simulink model "stellaris_helloworld"  (R2013a)
settings: Solver=FixedStepDiscrete  SolverMode=SingleTasking  StartTime=0.0  StopTime=10.0  FixedStep=0.2  RelTol=1e-3
libraries: stellaris_lib x4, simulink x2
settings Model: Creator=peselnikmg  LastModifiedBy=bas
settings OptimizationCC: ExpressionDepthLimit=2147483647  OptimizeModelRefInitCode=on  LifeSpan=1
settings DebuggingCC: UnderspecifiedInitializationDetection=Simplified  MergeDetectMultiDrivingBlocksExec=error  StrictBusMsg=ErrorOnBusTreatedAsVector  NonBusSignalsTreatedAsBus=error
settings HardwareCC: ProdEndianess=LittleEndian  ProdHWDeviceType=Texas Instruments->TMS470
settings RTWCC: SystemTargetFile=stellaris.tlc  TemplateMakefile=stellaris_tmf  PostCodeGenCommand=stellaris_customcode(buildInfo)  Description=TI Stellaris LaunchPad  GenerateReport=on  ProcessScript=stellaris_make_rtw_hook  IncludeHyperlinkInReport=on  GenerateTraceInfo=on  GenerateTraceReport=on  GenerateTraceReportSl=on  GenerateTraceReportSf=on  GenerateTraceReportEml=on  GenerateCodeMetricsReport=on  GenerateCodeReplacementReport=on
settings CodeAppCC: IgnoreCustomStorageClasses=off  CustomSymbolStrType=$N$R$M  InternalIdentifier=Classic
settings STFCustomTargetCC: CombineOutputUpdateFcns=on  ERTCustomFileBanners=on  SupportContinuousTime=off  SupportNonInlinedSFcns=off  MATLABClassNameForMDSCustomization=Simulink.SoftwareTarget.ERTCustomization  SystemTargetFile=stellaris.tlc
settings ERTTargetCC: GenerateSampleERTMain=off  ParMdlRefBuildCompliant=off  CompOptLevelCompliant=off  ConcurrentExecutionCompliant=off  ERTFirstTimeCompliant=off  ModelStepFunctionPrototypeControlCompliant=off  CPPClassGenCompliant=off  ERTCustomFileTemplate=stellaris_srmain.tlc

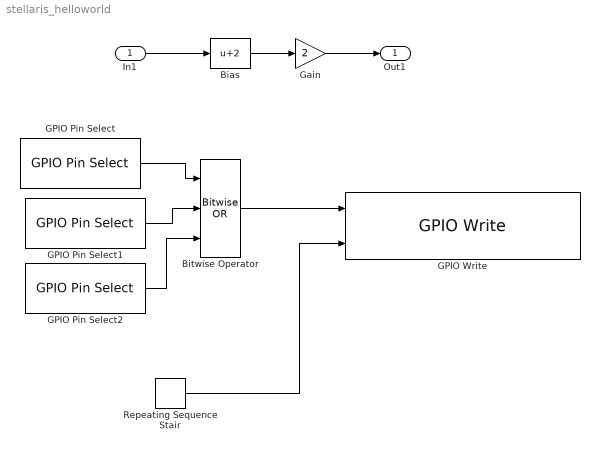
== system stellaris_helloworld ==
  In1 : Inport
  Bias : Bias  Bias=2
  Bitwise Operator : simulink/Logic and Bit Operations/Bitwise Operator  logicop=OR  UseBitMask=off  NumInputPorts=3  BitMask=bin2dec('11011001')  BitMaskRealWorld=Stored Integer
  GPIO Pin Select : stellaris_lib/GPIO/GPIO Pin Select  GPIO_PIN_X=GPIO_PIN_1
  GPIO Pin Select1 : stellaris_lib/GPIO/GPIO Pin Select  GPIO_PIN_X=GPIO_PIN_2
  GPIO Pin Select2 : stellaris_lib/GPIO/GPIO Pin Select  GPIO_PIN_X=GPIO_PIN_3
  GPIO Write : stellaris_lib/GPIO/GPIO Write  GPIO_PORTX_BASE=GPIO_PORTF_BASE
  Gain : Gain  Gain=2
  Repeating Sequence Stair : simulink/Sources/Repeating Sequence Stair  OutValues=[0 2 4 8].'  tsamp=1  OutMin=[]  OutMax=[]  OutDataTypeStr=uint8  OutputDataTypeScalingMode=uint8  OutDataType=fixdt(0,8)  ConRadixGroup=Best Precision: Vector-wise  OutScaling=2^-12
  Out1 : Outport
  wires:
  In1/1 -> Bias/1
  Bias/1 -> Gain/1
  Gain/1 -> Out1/1
  GPIO Pin Select1/1 -> Bitwise Operator/2
  GPIO Pin Select/1 -> Bitwise Operator/1
  GPIO Pin Select2/1 -> Bitwise Operator/3
  Bitwise Operator/1 -> GPIO Write/1
  Repeating Sequence Stair/1 -> GPIO Write/2
